simulink library "utils"  (R2023a)
settings: Solver=VariableStepAuto  StartTime=0.0  StopTime=10.0  RelTol=1e-3
settings Model: Creator=john  LastModifiedBy=john

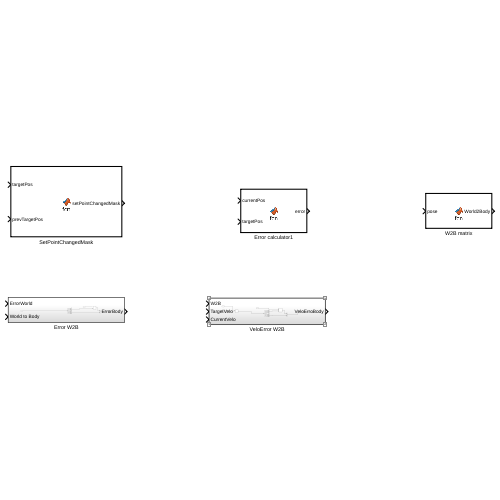
[thumbnail: Simulink's stored preview of the top-level diagram]
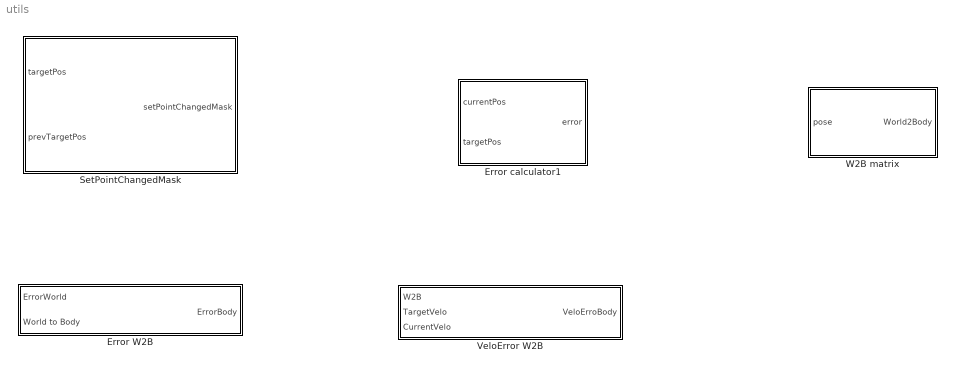
== system utils ==
  Error W2B : Subsystem
  Error calculator1 : MATLAB Function  TreatAsAtomicUnit=on
  SetPointChangedMask : MATLAB Function  TreatAsAtomicUnit=on
  VeloError W2B : Subsystem
  W2B matrix : MATLAB Function  TreatAsAtomicUnit=on

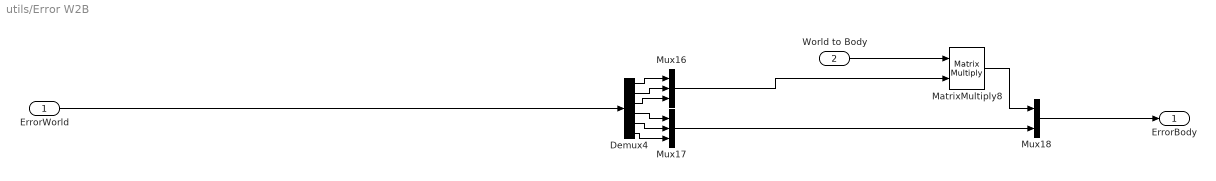
== system utils/Error W2B ==
  ErrorWorld : Inport
  World to Body : Inport  Port=2
  Demux4 : Demux  Outputs=6
  MatrixMultiply8 : Product  Multiplication=Matrix(*)
  Mux16 : Mux  Inputs=3
  Mux17 : Mux  Inputs=3
  Mux18 : Mux  Inputs=2
  ErrorBody : Outport
  wires:
  Demux4/2 -> Mux16/2
  Demux4/4 -> Mux17/1
  Mux16/1 -> MatrixMultiply8/2
  Demux4/6 -> Mux17/3
  Demux4/1 -> Mux16/1
  Demux4/5 -> Mux17/2
  Mux17/1 -> Mux18/2
  ErrorWorld/1 -> Demux4/1
  Demux4/3 -> Mux16/3
  MatrixMultiply8/1 -> Mux18/1
  Mux18/1 -> ErrorBody/1
  World to Body/1 -> MatrixMultiply8/1

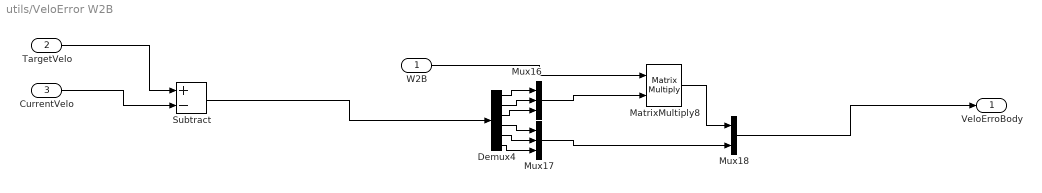
== system utils/VeloError W2B ==
  W2B : Inport
  TargetVelo : Inport  Port=2
  CurrentVelo : Inport  Port=3
  Demux4 : Demux  Outputs=6
  MatrixMultiply8 : Product  Multiplication=Matrix(*)
  Mux16 : Mux  Inputs=3
  Mux17 : Mux  Inputs=3
  Mux18 : Mux  Inputs=2
  Subtract : Sum  Inputs=+-
  VeloErroBody : Outport
  wires:
  TargetVelo/1 -> Subtract/1
  CurrentVelo/1 -> Subtract/2
  Demux4/2 -> Mux16/2
  Mux16/1 -> MatrixMultiply8/2
  Mux17/1 -> Mux18/2
  Demux4/6 -> Mux17/3
  Demux4/1 -> Mux16/1
  Demux4/4 -> Mux17/1
  Demux4/5 -> Mux17/2
  Demux4/3 -> Mux16/3
  MatrixMultiply8/1 -> Mux18/1
  Mux18/1 -> VeloErroBody/1
  Subtract/1 -> Demux4/1
  W2B/1 -> MatrixMultiply8/1

== matlab function utils/SetPointChangedMask ==
  data: targetPos input; setPointChangedMask output; prevTargetPos input
function setPointChangedMask = fcn(targetPos, prevTargetPos)

setPointChangedMask = zeros(6,1);
for i=1:6
    if(targetPos(i) ~= prevTargetPos(i))
        setPointChangedMask(i) = 1;
    else 
        setPointChangedMask(i) = 0;
    end
end

== matlab function utils/W2B matrix ==
  data: pose input; World2Body output
function World2Body= fcn(pose)

poseQuat = [pose(7), pose(4), pose(5), pose(6)];

World2Body = transpose(quat2rotm(poseQuat));

== matlab function utils/Error calculator1 ==
  data: currentPos input; targetPos input; error output
function error = fcn(currentPos, targetPos)

error = zeros(1,6);

%World Frame linear error
eWorld = zeros(1,3);

eWorld(1) = targetPos(1) - currentPos(1);
eWorld(2) = targetPos(2) - currentPos(2);
eWorld(3) = targetPos(3) - currentPos(3);

%Quaternion that represents position
currentQuat = [currentPos(7), currentPos(4), currentPos(5), currentPos(6)];

%make it a unit quaternion
unitQuat = currentQuat ./ norm(currentQuat);

%quaternion that we want to be at
setQuat = [targetPos(7), -targetPos(4), -targetPos(5), -targetPos(6)];

uSetQuat = setQuat ./ norm(setQuat);

%multiply the set quat by the conjugate of the unit quat to get an error
eQuat = quatmultiply(uSetQuat, conj(unitQuat));

%use shortest path
if(eQuat(1) < 0) 
    eQuat = -eQuat;
end


%total rotation angle
w = max(min(eQuat(1),1),-1);
theta = 2 * acos(w);

%s is sin(theta/2)
s = sqrt(max(1 - w^2,0));

%rotation axis and rotation vector
if s < 1e-6
   eRot = [0 0 0];
else
   axis = eQuat(2:4) / s;
   eRot = theta * axis;
end

theta_mag = norm(eRot);
if theta_mag < 1e-9
   axisError = [0 0 0];
else
   axisError = (sin(theta_mag/2)/theta_mag) * eRot;
end



error(1) = eWorld(1);
error(2) = eWorld(2);
error(3) = eWorld(3);
error(4) = -axisError(1);
error(5) = -axisError(2);
error(6) = -axisError(3);


end
